simulink model "data_mgmt"  (R2020a)
settings: Solver=VariableStepAuto  StartTime=0.0  StopTime=10.0  RelTol=1e-3
model workspace (MAT data in the model file):
  A = 2
  B = 2
settings Model: DataDictionary=new_data.sldd  OrderedModelArguments=off  Creator=Riyansh  LastModifiedBy=Riyansh

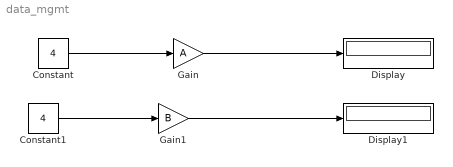
== system data_mgmt ==
  Constant : Constant  Value=4
  Constant1 : Constant  Value=4
  Display : Display
  Display1 : Display
  Gain : Gain  Gain=A
  Gain1 : Gain  Gain=B
  wires:
  Gain/1 -> Display/1
  Constant/1 -> Gain/1
  Gain1/1 -> Display1/1
  Constant1/1 -> Gain1/1
